simulink model "two_legged_raibert_hopper"  (R2014a)
settings: Solver=FixedStepDiscrete  StartTime=0.0  StopTime=inf  FixedStep=sample_time  RelTol=1e-3
undefined symbols (not defined in the file): boom_height, boom_mount_angle, boom_mount_to_center_diagonal, boom_mount_to_com, contact_threshold, control_start_time, desired_torso_angle, DiscIntNeverNeededParam, dt_thrust, dx_avg_desired, dx_avg_samples, dx_desired_step, extra_leg_damping, F_thrust, fcut_contact, g, i_limit_lateral, initial_dt, k_placement, k_sea, kd_flight, kd_lateral, kd_leg_angle, kd_leg_length_secondary, kd_torso, kd_virtual, ki_lateral, kp_flight_max, kp_flight_min, kp_lateral, kp_leg_angle, kp_leg_length_secondary, kp_torso, kp_virtual, l0_virtual, l_boom, l_max, l_min, l_retract, l_seg, lambda1, lambda2, lateral_offset, LEG_MTR_MAX_TORQUE, loaded_threshold, m_leg_motor, m_total_real, max_leg_angle, max_torque_lateral, min_leg_angle, sample_time, t_flight, x_limit
libraries: simulink x7
settings Model: xpc_rtwmakecfg_data=_xpcethercatlib_  BufferReuse=off  Creator=wmartin  LastModifiedBy=wmartin
settings SolverCC: EnableConcurrentExecution=on
settings DataIOCC: MaxDataPoints=1000000000  SaveFormat=StructureWithTime
settings OptimizationCC: BlockReduction=off  OptimizeBlockIOStorage=off  BufferReuse=off  GlobalBufferReuse=off  ExpressionFolding=off  ExpressionDepthLimit=2147483647  LocalBlockOutputs=off
settings DebuggingCC: UnderspecifiedInitializationDetection=Classic  StateNameClashWarn=warning
settings HardwareCC: ProdIntDivRoundTo=Zero  ProdEndianess=LittleEndian  ProdHWDeviceType=Generic->32-bit x86 compatible
settings RTWCC: SystemTargetFile=slrt.tlc  TemplateMakefile=slrt_default_tmf  Description=Simulink Real-Time  RTWVerbose=off  ProcessScript=slrt_make_rtw_hook  RTWCompilerOptimization=On
settings SimulinkRealTimeCC: GeneratePreprocessorConditionals=Disable all  EnableShiftOperators=on  RL32LogBufSizeModifier=100000000

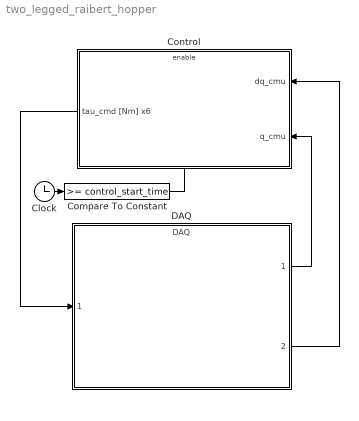
== system two_legged_raibert_hopper ==
  Clock : Clock
  Compare To Constant : simulink/Logic and Bit Operations/Compare To Constant  relop=>=  const=control_start_time  OutDataTypeStr=boolean
  Control : Subsystem
  DAQ : ModelReference  ModelNameDialog=DAQ  SimulationMode=Normal  ModelReferenceVersion=1.1405  CopyOfModelName=DAQ  DefaultDataLogging=on
  wires:
  DAQ/1 -> Control/2(q_cmu)
  DAQ/2 -> Control/1(dq_cmu)
  Clock/1 -> Compare To Constant/1
  Compare To Constant/1 -> Control/Enable
  Control/1(tau_cmd [Nm] x6) -> DAQ/1

== system two_legged_raibert_hopper/Control ==
  dq_cmu : Inport
  q_cmu : Inport  Port=2
  Enable : EnablePort  StatesWhenEnabling=reset
  Actuator Control : ModelReference  ModelNameDialog=Actuator_Control  SimulationMode=Normal  ModelReferenceVersion=1.2  CopyOfModelName=Actuator_Control  DefaultDataLogging=on
  Behavior Control : Subsystem
  tau_cmd [Nm] x6 : Outport  InitialOutput=[0 0 0 0 0 0]
  wires:
  Behavior Control/1(motor_torque_cmd) -> Actuator Control/1
  dq_cmu/1 -> Actuator Control/3, Behavior Control/1(dq_cmu)
  Actuator Control/1 -> tau_cmd [Nm] x6/1
  q_cmu/1 -> Actuator Control/2, Behavior Control/2(q_cmu)

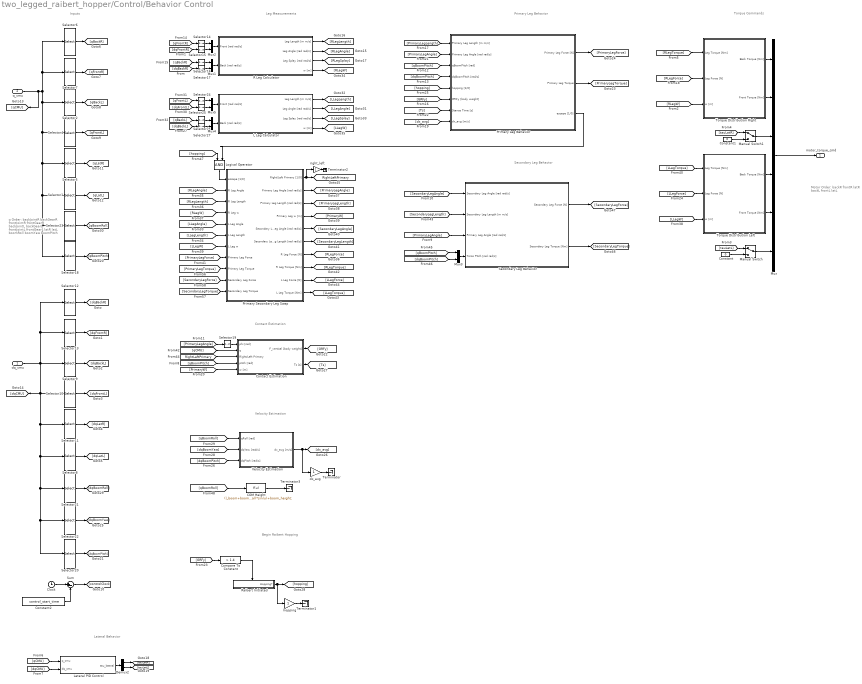
== system two_legged_raibert_hopper/Control/Behavior Control ==
  note: Motor Order:
      |
      | backR
      | frontR
      | latR
      | backL
      | frontL
      | latL
  note: q Order:
      |
      | backJointR
      | backGearR
      | frontJointR
      | frontGearR
      |
      | backJointL
      | backGearL
      | frontJointL
      | frontGearL
      |
      | latR
      | latL
      |
      | boomRoll
      | boomYaw
      | boomPitch
  note: Inputs
  note: Primary Leg Behavior
  note: Secondary Leg Behavior
  note: Torque Commands
  note: Lateral Behavior
  note: Leg Measurements
  note: Contact Estimation
  note: Velocity Estimation
  note: Begin Raibert Hopping
  dq_cmu : Inport
  q_cmu : Inport  Port=2
  COM Height : Fcn  Expr=(l_boom+boom_mount_to_center_diagonal)*sin(u)+boom_height;
  Clock : Clock
  Compare To Constant : simulink/Logic and Bit Operations/Compare To Constant  relop=>  const=1.4  OutDataTypeStr=boolean
  Constant : Constant  Value=0
  Constant1 : Constant  Value=0
  Constant2 : Constant  Value=control_start_time
  Contact Estimation : Subsystem
  Demux2 : Demux  Outputs=2
  L Leg Calculator : Subsystem
  Lateral PID Control : Subsystem
  Logical Operator : Logic  IconShape=distinctive  AllPortsSameDT=off  OutDataTypeStr=boolean
  Manual Switch : ManualSwitch
  Manual Switch1 : ManualSwitch
  Mux : Mux  Inputs=6
  Mux{1..5} (5 alike) : Mux  Inputs=2
  Primary Leg Behavior : Subsystem
  Primary Secondary Leg Swap : Subsystem
  R Leg Calculator : Subsystem
  Raibert Initiated : Subsystem
  Secondary Leg Behavior : Subsystem
  Selector1 : Selector  InputPortWidth=13  Indices=[10]
  Selector10 : Selector  InputPortWidth=13  Indices=[7 8]
  Selector11 : Selector  InputPortWidth=13  Indices=[9]
  Selector12 : Selector  InputPortWidth=13  Indices=[1 2]
  Selector13 : Selector  InputPortWidth=13  Indices=[3 4]
  Selector{14..17,19,24..27} (9 alike) : Selector  InputPortWidth=2  Indices=[1]
  Selector18 : Selector  InputPortWidth=13  Indices=[13]
  Selector2 : Selector  InputPortWidth=13  Indices=[5 6]
  Selector20 : Selector  InputPortWidth=13  Indices=[13]
  Selector21 : Selector  InputPortWidth=13  Indices=[11]
  Selector22 : Selector  InputPortWidth=13  Indices=[12]
  Selector23 : Selector  InputPortWidth=13  Indices=[11]
  Selector4 : Selector  InputPortWidth=13  Indices=[7 8]
  Selector5 : Selector  InputPortWidth=13  Indices=[9]
  Selector6 : Selector  InputPortWidth=13  Indices=[1 2]
  Selector7 : Selector  InputPortWidth=13  Indices=[3 4]
  Selector8 : Selector  InputPortWidth=13  Indices=[10]
  Selector9 : Selector  InputPortWidth=13  Indices=[5 6]
  Sum : Sum  Inputs=|+-
  Terminator{,1..3} (4 alike) : Terminator
  Torque Distribution Left : Subsystem
  Torque Distribution Right : Subsystem
  Velocity Estimation : Subsystem
  dx_avg : Gain
  hopping : Gain
  right_left : Gain
  motor_torque_cmd : Outport  OutputWhenDisabled=reset  InitialOutput=[0 0 0 0 0 0]
  tag scope: RightLeftPrimary=global
  wires:
  Lateral PID Control/1(tau_lateral) -> Demux2/1
  [dqCMU] -> Lateral PID Control/2(dq_cmu)
  [qCMU] -> Lateral PID Control/1(q_cmu)
  Sum/1 -> [controlClock]
  Selector4/1 -> [qFrontL]
  Selector2/1 -> [qBackL]
  Selector7/1 -> [qFrontR]
  Selector6/1 -> [qBackR]
  Selector1/1 -> [qLatL]
  Selector5/1 -> [qLatR]
  Constant2/1 -> Sum/2
  Clock/1 -> Sum/1
  Constant1/1 -> Manual Switch1/2
  Constant/1 -> Manual Switch/2
  Manual Switch/1 -> Mux/6
  Manual Switch1/1 -> Mux/3
  Mux/1 -> motor_torque_cmd/1
  Selector8/1 -> [dqLatL]
  Selector11/1 -> [dqLatR]
  Selector12/1 -> [dqBackR]
  Selector13/1 -> [dqFrontR]
  Selector9/1 -> [dqBackL]
  Selector10/1 -> [dqFrontL]
  [qBackR] -> Selector16/1
  [dqBackR] -> Selector17/1
  [qFrontR] -> Selector14/1
  [dqFrontR] -> Selector15/1
  Mux2/1 -> R Leg Calculator/1(Front [rad rad/s])
  Mux1/1 -> R Leg Calculator/2(Back [rad rad/s])
  R Leg Calculator/1("Leg Length [m m/s] ") -> [RLegLength]
  R Leg Calculator/2(Leg Angle [rad rad/s]) -> [RLegAngle]
  R Leg Calculator/3(Leg Splay [rad rad/s]) -> [RLegSplay]
  Torque Distribution Right/1(Back Torque [Nm]) -> Mux/1
  Torque Distribution Right/2(Front Torque [Nm]) -> Mux/2
  Demux2/1 -> [tauLatR]
  Demux2/2 -> [tauLatL]
  [tauLatR] -> Manual Switch1/1
  [tauLatL] -> Manual Switch/1
  [RLegW] -> Torque Distribution Right/3(w [m])
  Selector14/1 -> Mux2/1
  Selector15/1 -> Mux2/2
  Selector17/1 -> Mux1/2
  Selector16/1 -> Mux1/1
  [PrimaryW] -> Contact Estimation/5(w [m])
  q_cmu/1 -> Selector6/1, Selector7/1, Selector2/1, Selector4/1, Selector5/1, Selector18/1, Selector23/1, Selector1/1, [qCMU]
  Selector18/1 -> [qBoomPitch]
  [qBoomPitch] -> Contact Estimation/4(pitch [rad])
  [PrimaryLegAngle] -> Selector19/1
  Selector19/1 -> Contact Estimation/1(phi [rad])
  Contact Estimation/1(F_vertical [body weight]) -> [GRFy]
  Selector20/1 -> [dqBoomPitch]
  [RLegForce] -> Torque Distribution Right/2(Leg Force [N])
  [RLegTorque] -> Torque Distribution Right/1(Leg Torque [Nm])
  Selector22/1 -> [dqBoomYaw]
  Contact Estimation/2(Ts [s]) -> [Ts]
  [GRFy] -> Compare To Constant/1
  Raibert Initiated/1(Hopping?) -> hopping/1, [hopping]
  dq_cmu/1 -> Selector20/1, Selector22/1, Selector21/1, Selector8/1, Selector11/1, Selector10/1, [dqCMU], Selector12/1, Selector13/1, Selector9/1
  Selector21/1 -> [dqBoomRoll]
  Selector23/1 -> [qBoomRoll]
  [qBackL] -> Selector26/1
  [dqBackL] -> Selector27/1
  [qFrontL] -> Selector24/1
  [dqFrontL] -> Selector25/1
  Mux5/1 -> L Leg Calculator/1(Front [rad rad/s])
  Mux4/1 -> L Leg Calculator/2(Back [rad rad/s])
  L Leg Calculator/1("Leg Length [m m/s] ") -> [LLegLength]
  L Leg Calculator/2(Leg Angle [rad rad/s]) -> [LLegAngle]
  L Leg Calculator/3(Leg Splay [rad rad/s]) -> [LLegSplay]
  Selector24/1 -> Mux5/1
  Selector25/1 -> Mux5/2
  Selector27/1 -> Mux4/2
  Selector26/1 -> Mux4/1
  R Leg Calculator/4(w [m]) -> [RLegW]
  L Leg Calculator/4(w [m]) -> [LLegW]
  [LLegAngle] -> Primary Secondary Leg Swap/5(L Leg Angle)
  [LLegLength] -> Primary Secondary Leg Swap/6(L Leg Length)
  [LLegW] -> Primary Secondary Leg Swap/7(L Leg w)
  [RLegAngle] -> Primary Secondary Leg Swap/2(R Leg Angle)
  [RLegLength] -> Primary Secondary Leg Swap/3(R Leg Length)
  [RLegW] -> Primary Secondary Leg Swap/4(R Leg w)
  [PrimaryLegForce] -> Primary Secondary Leg Swap/8(Primary Leg Force)
  [PrimaryLegTorque] -> Primary Secondary Leg Swap/9(Primary Leg Torque)
  [SecondaryLegForce] -> Primary Secondary Leg Swap/10(Secondary Leg Force)
  [SecondaryLegTorque] -> Primary Secondary Leg Swap/11(Secondary Leg Torque)
  Primary Secondary Leg Swap/5(Secondary Leg Angle [rad rad/s]) -> [SecondaryLegAngle]
  Primary Secondary Leg Swap/6(Secondary Leg Length [rad rad/s]) -> [SecondaryLegLength]
  Primary Secondary Leg Swap/2(Primary Leg Angle [rad rad/s]) -> [PrimaryLegAngle]
  Primary Secondary Leg Swap/3(Primary Leg Length [rad rad/s]) -> [PrimaryLegLength]
  Primary Secondary Leg Swap/4(Primary Leg w [m]) -> [PrimaryW]
  Primary Secondary Leg Swap/7(R Leg Force [N]) -> [RLegForce]
  Primary Secondary Leg Swap/8(R Leg Torque [Nm]) -> [RLegTorque]
  Primary Secondary Leg Swap/9(L Leg Force [N]) -> [LLegForce]
  Primary Secondary Leg Swap/10(L Leg Torque [Nm]) -> [LLegTorque]
  Primary Leg Behavior/3(escape [1/0]) -> Logical Operator/2
  Primary Secondary Leg Swap/1(Right/Left Primary [1/0]) -> right_left/1, [RightLeftPrimary]
  [PrimaryLegLength] -> Primary Leg Behavior/1(Primary Leg Length [m m/s])
  [hopping] -> Primary Leg Behavior/5(hopping [1/0])
  [GRFy] -> Primary Leg Behavior/6(GRFy [body weight])
  [qBoomPitch] -> Primary Leg Behavior/3(qBoomPitch [rad])
  [dqBoomPitch] -> Primary Leg Behavior/4(dqBoomPitch [rad/s])
  [PrimaryLegAngle] -> Primary Leg Behavior/2(Primary Leg Angle [rad rad/s])
  [Ts] -> Primary Leg Behavior/7(Stance Time [s])
  [dx_avg] -> Primary Leg Behavior/8(dx_avg [m/s])
  Primary Leg Behavior/1(Primary Leg Force [N]) -> [PrimaryLegForce]
  Primary Leg Behavior/2(Primary Leg Torque) -> [PrimaryLegTorque]
  Velocity Estimation/1(dx_avg [m/s]) -> dx_avg/1, [dx_avg]
  [qBoomRoll] -> Velocity Estimation/1(qRoll [rad])
  [dqBoomYaw] -> Velocity Estimation/2(dqYaw [rad/s])
  [dqBoomPitch] -> Velocity Estimation/3(dqPitch [rad/s])
  dx_avg/1 -> Terminator/1
  hopping/1 -> Terminator1/1
  Torque Distribution Left/1(Back Torque [Nm]) -> Mux/4
  Torque Distribution Left/2(Front Torque [Nm]) -> Mux/5
  [LLegTorque] -> Torque Distribution Left/1(Leg Torque [Nm])
  [LLegForce] -> Torque Distribution Left/2(Leg Force [N])
  [LLegW] -> Torque Distribution Left/3(w [m])
  [qCMU] -> Contact Estimation/2(q)
  [RightLeftPrimary] -> Contact Estimation/3(Right/Left Primary)
  Secondary Leg Behavior/1(Secondary Leg Force [N]) -> [SecondaryLegForce]
  Secondary Leg Behavior/2(Secondary Leg Torque [Nm]) -> [SecondaryLegTorque]
  [PrimaryLegAngle] -> Secondary Leg Behavior/3(Primary Leg Angle [rad rad/s])
  [SecondaryLegAngle] -> Secondary Leg Behavior/1(Secondary Leg Angle [rad rad/s])
  [SecondaryLegLength] -> Secondary Leg Behavior/2(Secondary Leg Length [m m/s])
  [qBoomPitch] -> Mux3/1
  [dqBoomPitch] -> Mux3/2
  Mux3/1 -> Secondary Leg Behavior/4(Torso Pitch [rad rad/s])
  right_left/1 -> Terminator2/1
  [hopping] -> Logical Operator/1
  Logical Operator/1 -> Primary Secondary Leg Swap/1(escape [1/0])
  [qBoomRoll] -> COM Height/1
  COM Height/1 -> Terminator3/1
  Compare To Constant/1 -> Raibert Initiated/Enable

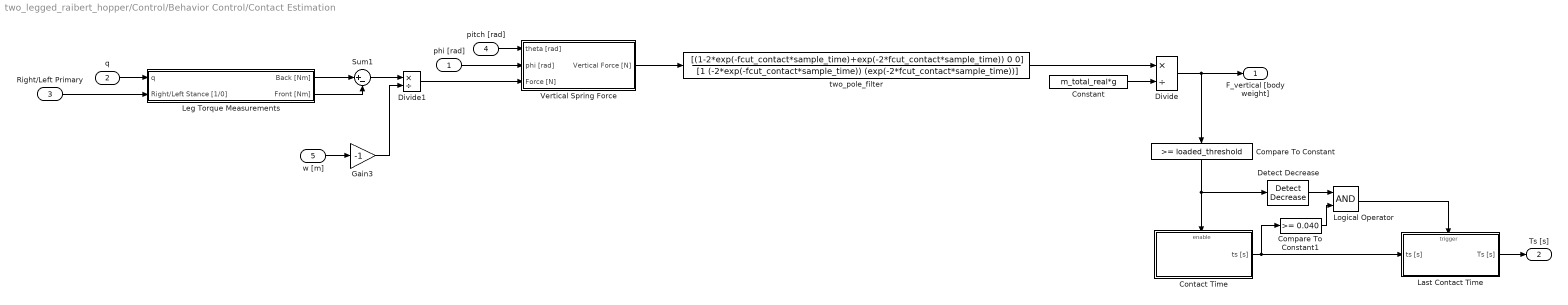
== system two_legged_raibert_hopper/Control/Behavior Control/Contact Estimation ==
  phi [rad] : Inport
  q : Inport  Port=2
  Right/Left Primary : Inport  Port=3
  pitch [rad] : Inport  Port=4
  w [m] : Inport  Port=5
  Compare To Constant : simulink/Logic and Bit Operations/Compare To Constant  relop=>=  const=loaded_threshold  OutDataTypeStr=boolean
  Compare To Constant1 : simulink/Logic and Bit Operations/Compare To Constant  relop=>=  const=0.040  OutDataTypeStr=boolean
  Constant : Constant  Value=m_total_real*g
  Contact Time : Subsystem
  Detect Decrease : simulink/Logic and Bit Operations/Detect Decrease  vinit=0.0  InputProcessing=Inherited  OutDataTypeStr=boolean
  Divide : Product  Inputs=*/
  Divide1 : Product  Inputs=*/
  Gain3 : Gain  Gain=-1
  Last Contact Time : Subsystem
  Leg Torque Measurements : Subsystem
  Logical Operator : Logic  AllPortsSameDT=off  OutDataTypeStr=boolean
  Sum1 : Sum  Inputs=|+-
  Vertical Spring Force : Subsystem
  two_pole_filter : DiscreteTransferFcn  Numerator=[(1-2*exp(-fcut_contact*sample_time)+exp(-2*fcut_contact*sample_time)) 0 0]  Denominator=[1 (-2*exp(-fcut_contact*sample_time)) (exp(-2*fcut_contact*sample_time))]  SampleTime=sample_time
  F_vertical [body weight] : Outport
  Ts [s] : Outport  Port=2
  wires:
  Vertical Spring Force/1(Vertical Force [N]) -> two_pole_filter/1
  Constant/1 -> Divide/2
  two_pole_filter/1 -> Divide/1
  q/1 -> Leg Torque Measurements/1(q)
  Leg Torque Measurements/1(Back [Nm]) -> Sum1/1
  Leg Torque Measurements/2(Front [Nm]) -> Sum1/2
  Sum1/1 -> Divide1/1
  Divide1/1 -> Vertical Spring Force/3(Force [N])
  pitch [rad]/1 -> Vertical Spring Force/1(theta [rad])
  w [m]/1 -> Gain3/1
  Gain3/1 -> Divide1/2
  phi [rad]/1 -> Vertical Spring Force/2(phi [rad])
  Last Contact Time/1(Ts [s]) -> Ts [s]/1
  Contact Time/1(ts [s]) -> Last Contact Time/1(ts [s]), Compare To Constant1/1
  Compare To Constant/1 -> Detect Decrease/1, Contact Time/Enable
  Divide/1 -> F_vertical [body weight]/1, Compare To Constant/1
  Logical Operator/1 -> Last Contact Time/Trigger
  Detect Decrease/1 -> Logical Operator/1
  Compare To Constant1/1 -> Logical Operator/2
  Right/Left Primary/1 -> Leg Torque Measurements/2(Right/Left Stance [1/0])

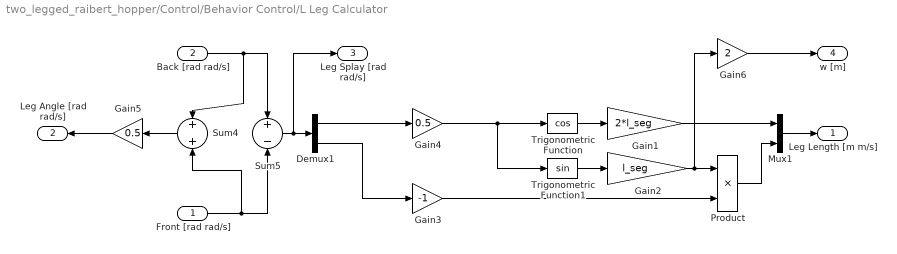
== system two_legged_raibert_hopper/Control/Behavior Control/L Leg Calculator ==
  Front [rad rad/s] : Inport
  Back [rad rad/s] : Inport  Port=2
  Demux1 : Demux  Outputs=2
  Gain1 : Gain  Gain=2*l_seg
  Gain2 : Gain  Gain=l_seg
  Gain3 : Gain  Gain=-1
  Gain4 : Gain  Gain=0.5
  Gain5 : Gain  Gain=0.5
  Gain6 : Gain  Gain=2
  Mux1 : Mux  Inputs=2
  Product : Product  RndMeth=Zero
  Sum4 : Sum  Inputs=+|+
  Sum5 : Sum  Inputs=+|-
  Trigonometric Function : Trigonometry  Operator=cos
  Trigonometric Function1 : Trigonometry
  "Leg Length [m m/s] " : Outport
  Leg Angle [rad rad/s] : Outport  Port=2
  Leg Splay [rad rad/s] : Outport  Port=3
  w [m] : Outport  Port=4
  wires:
  Gain5/1 -> Leg Angle [rad rad/s]/1
  Sum4/1 -> Gain5/1
  Mux1/1 -> "Leg Length [m m/s] "/1
  Sum5/1 -> Demux1/1, Leg Splay [rad rad/s]/1
  Gain2/1 -> Gain6/1, Product/1
  Demux1/1 -> Gain4/1
  Gain3/1 -> Product/2
  Demux1/2 -> Gain3/1
  Back [rad rad/s]/1 -> Sum5/1, Sum4/1
  Front [rad rad/s]/1 -> Sum4/2, Sum5/2
  Product/1 -> Mux1/2
  Trigonometric Function1/1 -> Gain2/1
  Gain1/1 -> Mux1/1
  Trigonometric Function/1 -> Gain1/1
  Gain4/1 -> Trigonometric Function/1, Trigonometric Function1/1
  Gain6/1 -> w [m]/1

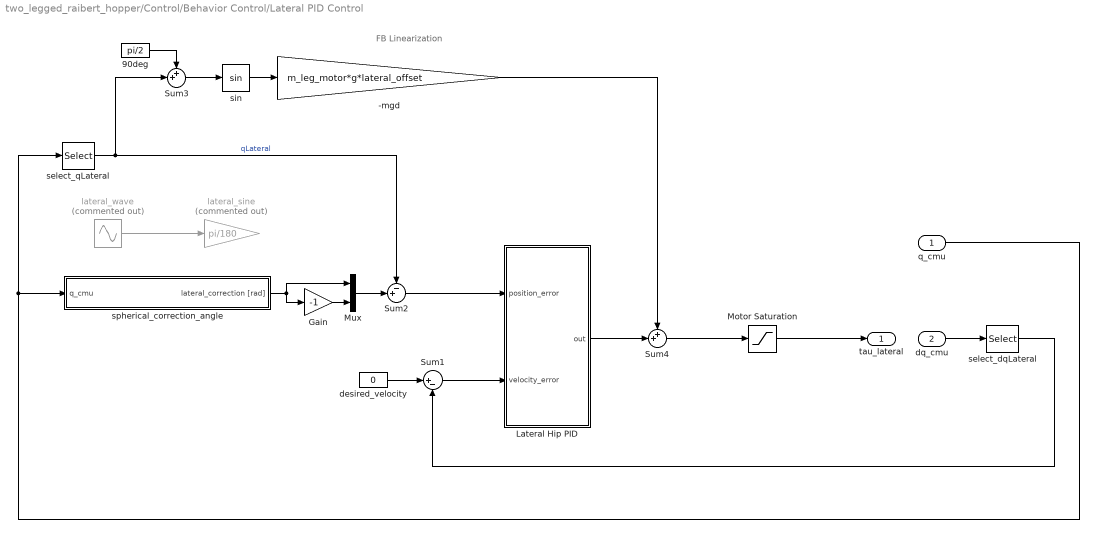
== system two_legged_raibert_hopper/Control/Behavior Control/Lateral PID Control ==
  note: FB Linearization
  q_cmu : Inport
  dq_cmu : Inport  Port=2
  -mgd : Gain  Gain=m_leg_motor*g*lateral_offset
  90deg : Constant  Value=pi/2
  Gain : Gain  Gain=-1
  Lateral Hip PID : Subsystem
  Motor Saturation : Saturate  UpperLimit=max_torque_lateral  LowerLimit=-max_torque_lateral
      settings: AttributesFormatString=Top: %<UpperLimit>\nBottom: %<LowerLimit>
  Mux : Mux  Inputs=2
  Sum1 : Sum  Inputs=|+-
  Sum2 : Sum  Inputs=-+|
  Sum3 : Sum  Inputs=++|
  Sum4 : Sum  Inputs=++|
  desired_velocity : Constant  Value=0
  lateral_sine : Gain  Commented=on  Gain=pi/180
  lateral_wave : Sin  Commented=on  Amplitude=5  Frequency=2*pi*(1/2)  SampleTime=0
  select_dqLateral : Selector  InputPortWidth=13  Indices=[9 10]
  select_qLateral : Selector  InputPortWidth=13  Indices=[9 10]
  sin : Trigonometry
  spherical_correction_angle : Subsystem
  tau_lateral : Outport
  wires:
  lateral_wave/1 -> lateral_sine/1
  Lateral Hip PID/1(out) -> Sum4/2
  Sum2/1 -> Lateral Hip PID/1(position_error)
  q_cmu/1 -> spherical_correction_angle/1(q_cmu), select_qLateral/1
  select_dqLateral/1 -> Sum1/2
  dq_cmu/1 -> select_dqLateral/1
  Sum4/1 -> Motor Saturation/1
  desired_velocity/1 -> Sum1/1
  Sum1/1 -> Lateral Hip PID/2(velocity_error)
  Gain/1 -> Mux/2
  Mux/1 -> Sum2/2
  select_qLateral/1 -> Sum3/2, Sum2/1  "qLateral"
  Motor Saturation/1 -> tau_lateral/1
  spherical_correction_angle/1(lateral_correction [rad]) -> Mux/1, Gain/1
  -mgd/1 -> Sum4/1
  Sum3/1 -> sin/1
  90deg/1 -> Sum3/1
  sin/1 -> -mgd/1

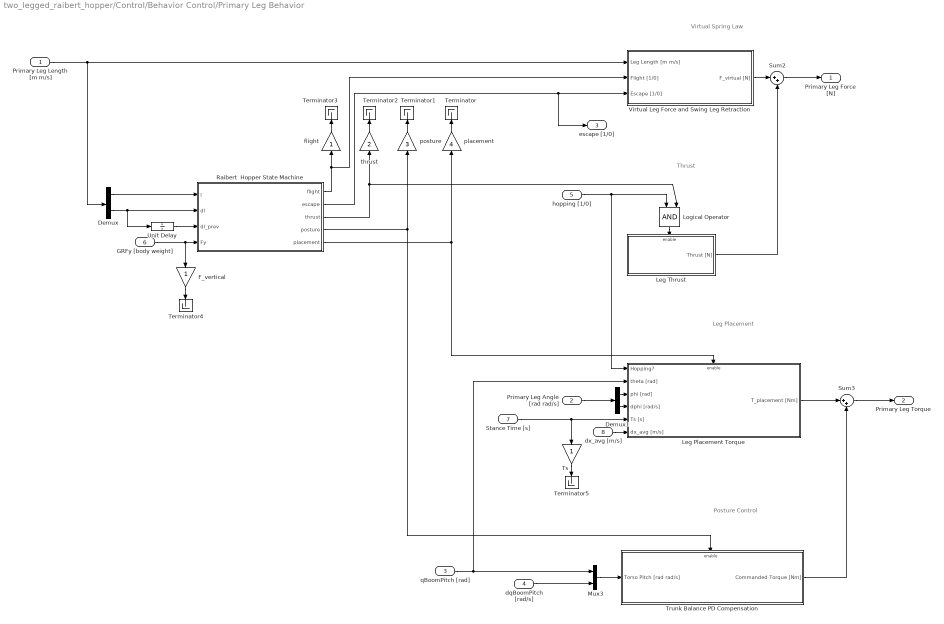
== system two_legged_raibert_hopper/Control/Behavior Control/Primary Leg Behavior ==
  note: Virtual Spring Law
  note: Thrust
  note: Posture Control
  note: Leg Placement
  Primary Leg Length [m m/s] : Inport
  Primary Leg Angle [rad rad/s] : Inport  Port=2
  qBoomPitch [rad] : Inport  Port=3
  dqBoomPitch [rad/s] : Inport  Port=4
  hopping [1/0] : Inport  Port=5
  GRFy [body weight] : Inport  Port=6
  Stance Time [s] : Inport  Port=7
  dx_avg [m/s] : Inport  Port=8
  Demux : Demux  Outputs=2
  Demux1 : Demux  Outputs=2
  F_vertical : Gain
  Leg Placement Torque : Subsystem
  Leg Thrust : Subsystem
  Logical Operator : Logic  IconShape=distinctive  AllPortsSameDT=off  OutDataTypeStr=boolean
  Mux3 : Mux  Inputs=2
  Raibert  Hopper State Machine : State Transition Table  TreatAsAtomicUnit=on
  Sum2 : Sum  Inputs=|++
  Sum3 : Sum  Inputs=|++
  Terminator{,1..5} (6 alike) : Terminator
  Trunk Balance PD Compensation : Subsystem
  Ts : Gain
  Unit Delay : UnitDelay  SampleTime=-1
  Virtual Leg Force and Swing Leg Retraction : Subsystem
  flight : Gain
  placement : Gain  Gain=4
  posture : Gain  Gain=3
  thrust : Gain  Gain=2
  Primary Leg Force [N] : Outport
  Primary Leg Torque : Outport  Port=2
  escape [1/0] : Outport  Port=3
  wires:
  Raibert  Hopper State Machine/4(posture) -> Trunk Balance PD Compensation/Enable, posture/1
  Mux3/1 -> Trunk Balance PD Compensation/1(Torso Pitch [rad rad/s])
  qBoomPitch [rad]/1 -> Mux3/1, Leg Placement Torque/2(theta [rad])
  dqBoomPitch [rad/s]/1 -> Mux3/2
  Trunk Balance PD Compensation/1(Commanded Torque [Nm]) -> Sum3/2
  Unit Delay/1 -> Raibert  Hopper State Machine/3(dl_prev)
  GRFy [body weight]/1 -> F_vertical/1, Raibert  Hopper State Machine/4(Fy)
  Demux/2 -> Unit Delay/1, Raibert  Hopper State Machine/2(dl)
  Raibert  Hopper State Machine/3(thrust) -> Logical Operator/2, thrust/1
  Leg Thrust/1(Thrust [N]) -> Sum2/2
  Sum2/1 -> Primary Leg Force [N]/1
  Raibert  Hopper State Machine/1(flight) -> flight/1, Virtual Leg Force and Swing Leg Retraction/2(Flight [1/0])
  Virtual Leg Force and Swing Leg Retraction/1(F_virtual [N]) -> Sum2/1
  Raibert  Hopper State Machine/2(escape) -> escape [1/0]/1, Virtual Leg Force and Swing Leg Retraction/3(Escape [1/0])
  Leg Placement Torque/1(T_placement [Nm]) -> Sum3/1
  Sum3/1 -> Primary Leg Torque/1
  dx_avg [m/s]/1 -> Leg Placement Torque/6(dx_avg [m/s])
  Demux1/1 -> Leg Placement Torque/3(phi [rad])
  Demux1/2 -> Leg Placement Torque/4(dphi [rad/s])
  Primary Leg Angle [rad rad/s]/1 -> Demux1/1
  Stance Time [s]/1 -> Leg Placement Torque/5(Ts [s]), Ts/1
  Raibert  Hopper State Machine/5(placement) -> Leg Placement Torque/Enable, placement/1
  Logical Operator/1 -> Leg Thrust/Enable
  placement/1 -> Terminator/1
  posture/1 -> Terminator1/1
  thrust/1 -> Terminator2/1
  Primary Leg Length [m m/s]/1 -> Demux/1, Virtual Leg Force and Swing Leg Retraction/1(Leg Length [m m/s])
  F_vertical/1 -> Terminator4/1
  flight/1 -> Terminator3/1
  Demux/1 -> Raibert  Hopper State Machine/1(l)
  Ts/1 -> Terminator5/1
  hopping [1/0]/1 -> Leg Placement Torque/1(Hopping?), Logical Operator/1

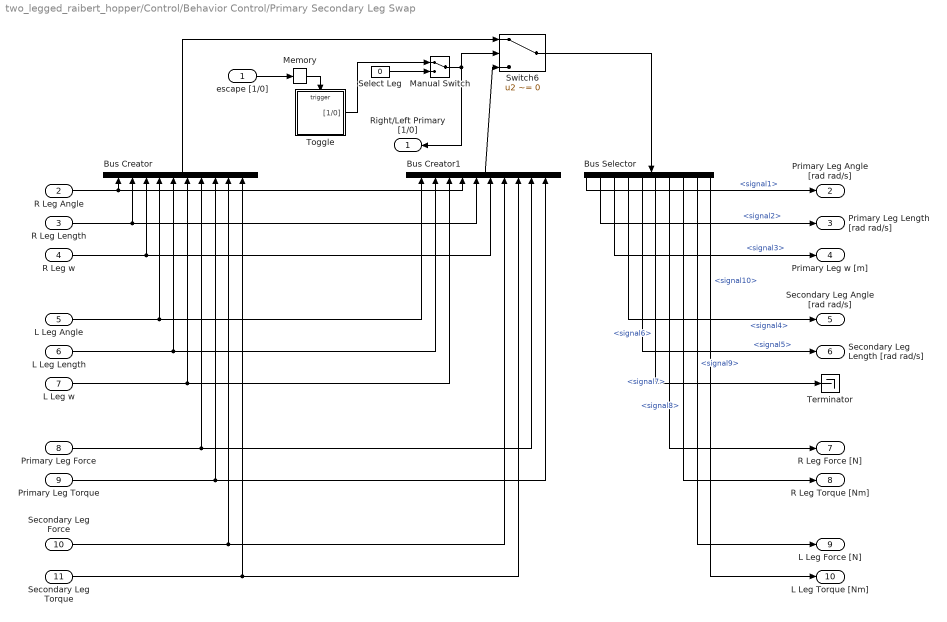
== system two_legged_raibert_hopper/Control/Behavior Control/Primary Secondary Leg Swap ==
  escape [1/0] : Inport
  R Leg Angle : Inport  Port=2
  R Leg Length : Inport  Port=3
  R Leg w : Inport  Port=4
  L Leg Angle : Inport  Port=5
  L Leg Length : Inport  Port=6
  L Leg w : Inport  Port=7
  Primary Leg Force : Inport  Port=8
  Primary Leg Torque : Inport  Port=9
  Secondary Leg Force : Inport  Port=10
  Secondary Leg Torque : Inport  Port=11
  Bus Creator : BusCreator  Inputs=10
  Bus Creator1 : BusCreator  Inputs=10
  Bus Selector : BusSelector  OutputSignals=signal1,signal2,signal3,signal4,signal5,signal6,signal7,signal8,signal9,signal10
  Manual Switch : ManualSwitch
  Memory : Memory  InheritSampleTime=on
  Select Leg : Constant  Value=0  OutDataTypeStr=boolean
  Switch6 : Switch  Criteria=u2 ~= 0  ZeroCross=off
  Terminator : Terminator
  Toggle : Subsystem
  Right/Left Primary [1/0] : Outport
  Primary Leg Angle [rad rad/s] : Outport  Port=2
  Primary Leg Length [rad rad/s] : Outport  Port=3
  Primary Leg w [m] : Outport  Port=4
  Secondary Leg Angle [rad rad/s] : Outport  Port=5
  Secondary Leg Length [rad rad/s] : Outport  Port=6
  R Leg Force [N] : Outport  Port=7
  R Leg Torque [Nm] : Outport  Port=8
  L Leg Force [N] : Outport  Port=9
  L Leg Torque [Nm] : Outport  Port=10
  wires:
  Switch6/1 -> Bus Selector/1
  Bus Creator1/1 -> Switch6/3
  Bus Creator/1 -> Switch6/1
  Primary Leg Torque/1 -> Bus Creator1/10, Bus Creator/8
  Secondary Leg Torque/1 -> Bus Creator1/8, Bus Creator/10
  Secondary Leg Force/1 -> Bus Creator1/7, Bus Creator/9
  escape [1/0]/1 -> Memory/1
  R Leg Length/1 -> Bus Creator1/5, Bus Creator/2
  L Leg w/1 -> Bus Creator/6, Bus Creator1/3
  R Leg Angle/1 -> Bus Creator1/4, Bus Creator/1
  R Leg w/1 -> Bus Creator1/6, Bus Creator/3
  Primary Leg Force/1 -> Bus Creator1/9, Bus Creator/7
  L Leg Length/1 -> Bus Creator/5, Bus Creator1/2
  L Leg Angle/1 -> Bus Creator/4, Bus Creator1/1
  Bus Selector/1 -> Primary Leg Angle [rad rad/s]/1  "<signal1>"
  Bus Selector/2 -> Primary Leg Length [rad rad/s]/1  "<signal2>"
  Bus Selector/3 -> Primary Leg w [m]/1  "<signal3>"
  Bus Selector/4 -> Secondary Leg Angle [rad rad/s]/1  "<signal4>"
  Bus Selector/5 -> Secondary Leg Length [rad rad/s]/1  "<signal5>"
  Bus Selector/6 -> Terminator/1  "<signal6>"
  Bus Selector/7 -> R Leg Force [N]/1  "<signal7>"
  Bus Selector/8 -> R Leg Torque [Nm]/1  "<signal8>"
  Bus Selector/9 -> L Leg Force [N]/1  "<signal9>"
  Bus Selector/10 -> L Leg Torque [Nm]/1  "<signal10>"
  Select Leg/1 -> Manual Switch/2
  Manual Switch/1 -> Switch6/2, Right/Left Primary [1/0]/1
  Toggle/1("[1/0]") -> Manual Switch/1
  Memory/1 -> Toggle/Trigger

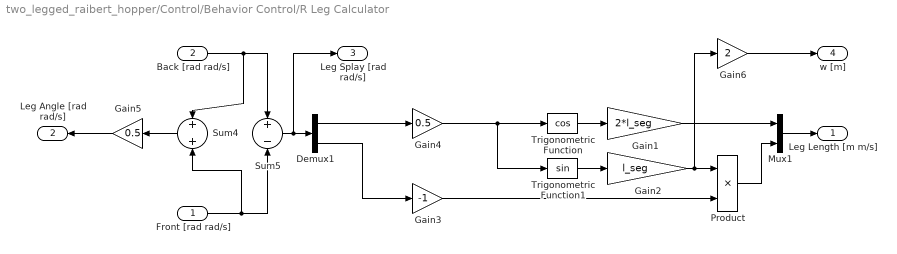
== system two_legged_raibert_hopper/Control/Behavior Control/R Leg Calculator ==
  Front [rad rad/s] : Inport
  Back [rad rad/s] : Inport  Port=2
  Demux1 : Demux  Outputs=2
  Gain1 : Gain  Gain=2*l_seg
  Gain2 : Gain  Gain=l_seg
  Gain3 : Gain  Gain=-1
  Gain4 : Gain  Gain=0.5
  Gain5 : Gain  Gain=0.5
  Gain6 : Gain  Gain=2
  Mux1 : Mux  Inputs=2
  Product : Product  RndMeth=Zero
  Sum4 : Sum  Inputs=+|+
  Sum5 : Sum  Inputs=+|-
  Trigonometric Function : Trigonometry  Operator=cos
  Trigonometric Function1 : Trigonometry
  "Leg Length [m m/s] " : Outport
  Leg Angle [rad rad/s] : Outport  Port=2
  Leg Splay [rad rad/s] : Outport  Port=3
  w [m] : Outport  Port=4
  wires:
  Gain6/1 -> w [m]/1
  Gain4/1 -> Trigonometric Function1/1, Trigonometric Function/1
  Trigonometric Function/1 -> Gain1/1
  Gain1/1 -> Mux1/1
  Trigonometric Function1/1 -> Gain2/1
  Product/1 -> Mux1/2
  Front [rad rad/s]/1 -> Sum5/2, Sum4/2
  Back [rad rad/s]/1 -> Sum4/1, Sum5/1
  Demux1/2 -> Gain3/1
  Gain3/1 -> Product/2
  Demux1/1 -> Gain4/1
  Gain2/1 -> Product/1, Gain6/1
  Sum5/1 -> Leg Splay [rad rad/s]/1, Demux1/1
  Mux1/1 -> "Leg Length [m m/s] "/1
  Sum4/1 -> Gain5/1
  Gain5/1 -> Leg Angle [rad rad/s]/1

== system two_legged_raibert_hopper/Control/Behavior Control/Raibert Initiated ==
  Enable : EnablePort  StatesWhenEnabling=reset
  Constant : Constant
  Hopping? : Outport  InitialOutput=[0]
  wires:
  Constant/1 -> Hopping?/1

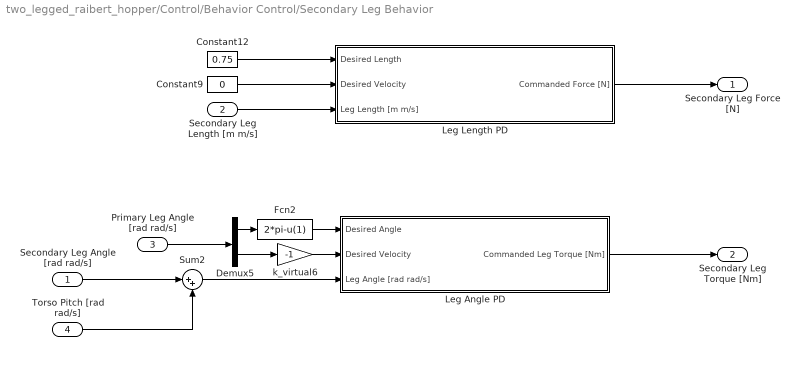
== system two_legged_raibert_hopper/Control/Behavior Control/Secondary Leg Behavior ==
  Secondary Leg Angle [rad rad/s] : Inport
  Secondary Leg Length [m m/s] : Inport  Port=2
  Primary Leg Angle [rad rad/s] : Inport  Port=3
  Torso Pitch [rad rad/s] : Inport  Port=4
  Constant12 : Constant  Value=0.75
  Constant9 : Constant  Value=0
  Demux5 : Demux  Outputs=2
  Fcn2 : Fcn  Expr=2*pi-u(1)
  Leg Angle PD : Subsystem
  Leg Length PD : Subsystem
  Sum2 : Sum  Inputs=|++
  k_virtual6 : Gain  Gain=-1
  Secondary Leg Force [N] : Outport
  Secondary Leg Torque [Nm] : Outport  Port=2
  wires:
  Constant9/1 -> Leg Length PD/2(Desired Velocity)
  Constant12/1 -> Leg Length PD/1(Desired Length)
  Secondary Leg Length [m m/s]/1 -> Leg Length PD/3(Leg Length [m m/s])
  Leg Length PD/1(Commanded Force [N]) -> Secondary Leg Force [N]/1
  Secondary Leg Angle [rad rad/s]/1 -> Sum2/1
  Torso Pitch [rad rad/s]/1 -> Sum2/2
  Sum2/1 -> Leg Angle PD/3(Leg Angle [rad rad/s])
  Fcn2/1 -> Leg Angle PD/1(Desired Angle)
  k_virtual6/1 -> Leg Angle PD/2(Desired Velocity)
  Primary Leg Angle [rad rad/s]/1 -> Demux5/1
  Demux5/1 -> Fcn2/1
  Demux5/2 -> k_virtual6/1
  Leg Angle PD/1(Commanded Leg Torque [Nm]) -> Secondary Leg Torque [Nm]/1

== system two_legged_raibert_hopper/Control/Behavior Control/Torque Distribution Left ==
  Leg Torque [Nm] : Inport
  Leg Force [N] : Inport  Port=2
  w [m] : Inport  Port=3
  Gain : Gain  Gain=0.5
  Gain1 : Gain  Gain=0.5
  Motor Torque Saturation Optimization : MATLAB Function  TreatAsAtomicUnit=on
  Product : Product  RndMeth=Zero
  Sum : Sum  Inputs=|++
  Sum1 : Sum  Inputs=+-|
  Back Torque [Nm] : Outport
  Front Torque [Nm] : Outport  Port=2
  wires:
  Gain/1 -> Motor Torque Saturation Optimization/1(x1s)
  Gain1/1 -> Motor Torque Saturation Optimization/2(x2s)
  Product/1 -> Gain1/1
  Leg Force [N]/1 -> Product/1
  Motor Torque Saturation Optimization/2(t2) -> Sum/2, Sum1/2
  w [m]/1 -> Product/2
  Motor Torque Saturation Optimization/1(t1) -> Sum1/1, Sum/1
  Sum/1 -> Front Torque [Nm]/1
  Leg Torque [Nm]/1 -> Gain/1
  Sum1/1 -> Back Torque [Nm]/1

== system two_legged_raibert_hopper/Control/Behavior Control/Torque Distribution Right ==
  Leg Torque [Nm] : Inport
  Leg Force [N] : Inport  Port=2
  w [m] : Inport  Port=3
  Gain : Gain  Gain=0.5
  Gain1 : Gain  Gain=0.5
  Motor Torque Saturation Optimization : MATLAB Function  TreatAsAtomicUnit=on
  Product : Product  RndMeth=Zero
  Sum : Sum  Inputs=|++
  Sum1 : Sum  Inputs=+-|
  Back Torque [Nm] : Outport
  Front Torque [Nm] : Outport  Port=2
  wires:
  Sum1/1 -> Back Torque [Nm]/1
  Leg Torque [Nm]/1 -> Gain/1
  Sum/1 -> Front Torque [Nm]/1
  Motor Torque Saturation Optimization/1(t1) -> Sum/1, Sum1/1
  w [m]/1 -> Product/2
  Motor Torque Saturation Optimization/2(t2) -> Sum1/2, Sum/2
  Leg Force [N]/1 -> Product/1
  Product/1 -> Gain1/1
  Gain1/1 -> Motor Torque Saturation Optimization/2(x2s)
  Gain/1 -> Motor Torque Saturation Optimization/1(x1s)

== system two_legged_raibert_hopper/Control/Behavior Control/Velocity Estimation ==
  qRoll [rad] : Inport
  dqYaw [rad/s] : Inport  Port=2
  dqPitch [rad/s] : Inport  Port=3
  Recursive Moving Average : Subsystem
  dx_from_yaw_and_roll : MATLAB Function  TreatAsAtomicUnit=on
  dx_avg [m/s] : Outport
  wires:
  Recursive Moving Average/1(dx_avg [m/s]) -> dx_avg [m/s]/1
  dx_from_yaw_and_roll/1(dx) -> Recursive Moving Average/1(dx [m/s])
  dqYaw [rad/s]/1 -> dx_from_yaw_and_roll/2(dqYaw)
  qRoll [rad]/1 -> dx_from_yaw_and_roll/1(qRoll)
  dqPitch [rad/s]/1 -> dx_from_yaw_and_roll/3(dqPitch)

== system two_legged_raibert_hopper/Control/Behavior Control/Contact Estimation/Contact Time ==
  Enable : EnablePort  StatesWhenEnabling=reset  ShowOutputPort=on
  Constant : Constant
  Discrete-Time Integrator : DiscreteIntegrator  IntegratorMethod=Accumulation: Forward Euler  gainval=sample_time  ExternalReset=rising  SampleTime=sample_time  ICPrevOutput=DiscIntNeverNeededParam  ICPrevScaledInput=DiscIntNeverNeededParam
  ts [s] : Outport  InitialOutput=[0]
  wires:
  Constant/1 -> Discrete-Time Integrator/1
  Enable/1 -> Discrete-Time Integrator/2
  Discrete-Time Integrator/1 -> ts [s]/1

== system two_legged_raibert_hopper/Control/Behavior Control/Contact Estimation/Last Contact Time ==
  ts [s] : Inport
  Trigger : TriggerPort  TriggerType=falling  PortDimensions=1
  Ts [s] : Outport  InitialOutput=[initial_dt]
  wires:
  ts [s]/1 -> Ts [s]/1

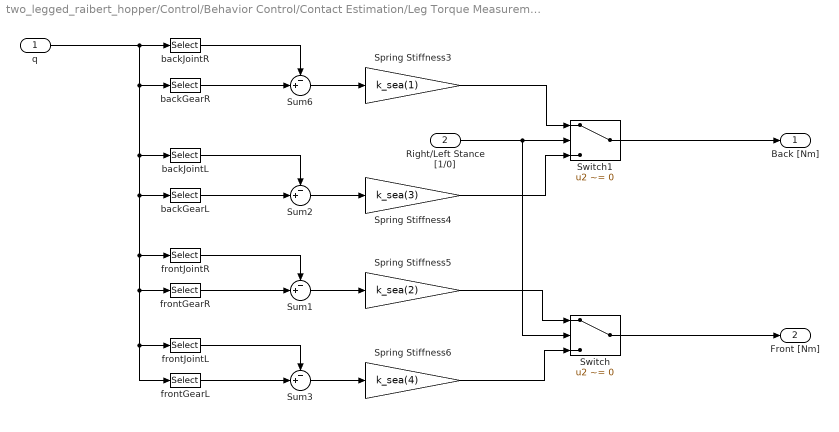
== system two_legged_raibert_hopper/Control/Behavior Control/Contact Estimation/Leg Torque Measurements ==
  q : Inport
  Right/Left Stance [1/0] : Inport  Port=2
  Spring Stiffness3 : Gain  Gain=k_sea(1)
  Spring Stiffness4 : Gain  Gain=k_sea(3)
  Spring Stiffness5 : Gain  Gain=k_sea(2)
  Spring Stiffness6 : Gain  Gain=k_sea(4)
  Sum{1..3,6} (4 alike) : Sum  Inputs=-+|
  Switch : Switch  Criteria=u2 ~= 0
  Switch1 : Switch  Criteria=u2 ~= 0
  backGearL : Selector  InputPortWidth=13  Indices=[6]
  backGearR : Selector  InputPortWidth=13  Indices=[2]
  backJointL : Selector  InputPortWidth=13  Indices=[5]
  backJointR : Selector  InputPortWidth=13  Indices=[1]
  frontGearL : Selector  InputPortWidth=13  Indices=[8]
  frontGearR : Selector  InputPortWidth=13  Indices=[4]
  frontJointL : Selector  InputPortWidth=13  Indices=[7]
  frontJointR : Selector  InputPortWidth=13  Indices=[3]
  Back [Nm] : Outport
  Front [Nm] : Outport  Port=2
  wires:
  Right/Left Stance [1/0]/1 -> Switch1/2, Switch/2
  Sum3/1 -> Spring Stiffness6/1
  Sum2/1 -> Spring Stiffness4/1
  Switch1/1 -> Back [Nm]/1
  backJointL/1 -> Sum2/1
  frontGearL/1 -> Sum3/2
  frontJointL/1 -> Sum3/1
  backGearL/1 -> Sum2/2
  Sum6/1 -> Spring Stiffness3/1
  Sum1/1 -> Spring Stiffness5/1
  Switch/1 -> Front [Nm]/1
  backJointR/1 -> Sum6/1
  frontGearR/1 -> Sum1/2
  frontJointR/1 -> Sum1/1
  backGearR/1 -> Sum6/2
  q/1 -> backGearR/1, backJointL/1, backGearL/1, frontJointR/1, frontGearR/1, frontJointL/1, frontGearL/1, backJointR/1
  Spring Stiffness3/1 -> Switch1/1
  Spring Stiffness4/1 -> Switch1/3
  Spring Stiffness5/1 -> Switch/1
  Spring Stiffness6/1 -> Switch/3

== system two_legged_raibert_hopper/Control/Behavior Control/Contact Estimation/Vertical Spring Force ==
  theta [rad] : Inport
  phi [rad] : Inport  Port=2
  Force [N] : Inport  Port=3
  Gain : Gain  Gain=-1
  Product : Product
  Sum : Sum  Inputs=++|
  Trigonometric Function : Trigonometry  Operator=cos
  Vertical Force [N] : Outport
  wires:
  Force [N]/1 -> Product/1
  phi [rad]/1 -> Sum/2
  theta [rad]/1 -> Sum/1
  Trigonometric Function/1 -> Product/2
  Product/1 -> Gain/1
  Sum/1 -> Trigonometric Function/1
  Gain/1 -> Vertical Force [N]/1

== system two_legged_raibert_hopper/Control/Behavior Control/Lateral PID Control/Lateral Hip PID ==
  position_error : Inport
  velocity_error : Inport  Port=2
  Discrete-Time Integrator : DiscreteIntegrator  IntegratorMethod=Integration: Trapezoidal  SampleTime=sample_time  LimitOutput=on  UpperSaturationLimit=i_limit_lateral  LowerSaturationLimit=-i_limit_lateral  ICPrevOutput=DiscIntNeverNeededParam  ICPrevScaledInput=DiscIntNeverNeededParam
  Sum : Sum  Inputs=+++
  kd_lateral : Gain  Description=xPCTag(1)=kd_lateral;  Gain=kd_lateral
  ki_lateral : Gain  Description=xPCTag(1)=ki_lateral;  Gain=ki_lateral
  kp_lateral : Gain  Description=xPCTag(1)=kp_lateral;  Gain=kp_lateral
  out : Outport
  wires:
  velocity_error/1 -> kd_lateral/1
  Discrete-Time Integrator/1 -> Sum/3
  ki_lateral/1 -> Discrete-Time Integrator/1
  kp_lateral/1 -> Sum/2
  position_error/1 -> ki_lateral/1, kp_lateral/1
  Sum/1 -> out/1
  kd_lateral/1 -> Sum/1

== system two_legged_raibert_hopper/Control/Behavior Control/Lateral PID Control/spherical_correction_angle ==
  q_cmu : Inport
  Selector : Selector  InputPortWidth=13  Indices=[11]
  Sum1 : Sum  Inputs=|+-
  Terminator2 : Terminator
  boom_mount_angle : Constant  Value=boom_mount_angle
  lateral_correction : Gain  Gain=180/pi
  lateral_correction [rad] : Outport
  wires:
  Sum1/1 -> lateral_correction/1, lateral_correction [rad]/1
  Selector/1 -> Sum1/1  "qBoomRoll"
  q_cmu/1 -> Selector/1
  boom_mount_angle/1 -> Sum1/2
  lateral_correction/1 -> Terminator2/1

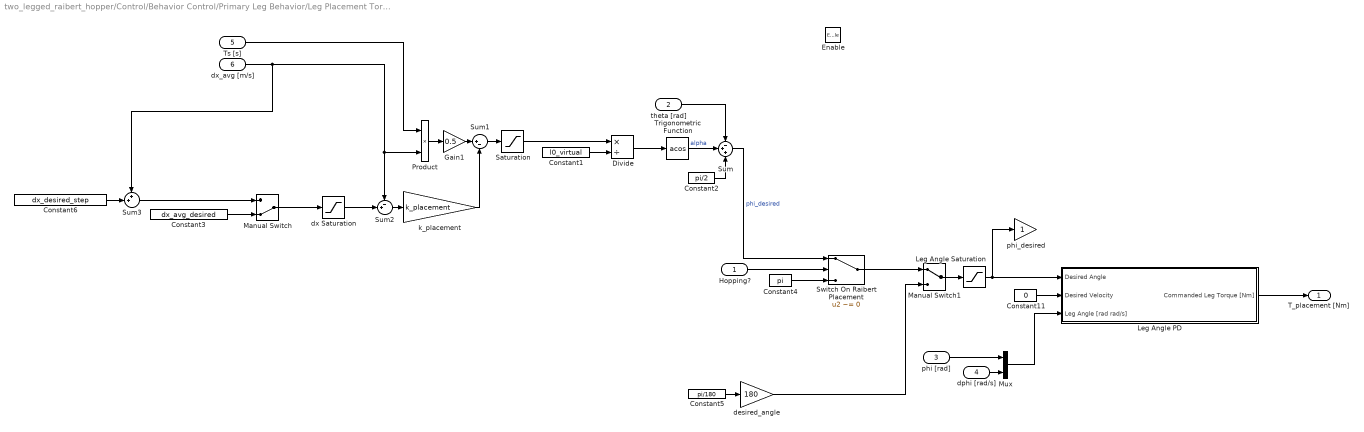
== system two_legged_raibert_hopper/Control/Behavior Control/Primary Leg Behavior/Leg Placement Torque ==
  Hopping? : Inport
  theta [rad] : Inport  Port=2
  phi [rad] : Inport  Port=3
  dphi [rad/s] : Inport  Port=4
  Ts [s] : Inport  Port=5
  dx_avg [m/s] : Inport  Port=6
  Enable : EnablePort  StatesWhenEnabling=reset
  Constant1 : Constant  Value=l0_virtual
  Constant11 : Constant  Value=0
  Constant2 : Constant  Value=pi/2
  Constant3 : Constant  Value=dx_avg_desired
  Constant4 : Constant  Value=pi
  Constant5 : Constant  Value=pi/180
  Constant6 : Constant  Value=dx_desired_step
  Divide : Product  Inputs=*/
  Gain1 : Gain  Gain=0.5
  Leg Angle PD : Subsystem
  Leg Angle Saturation : Saturate  UpperLimit=max_leg_angle  LowerLimit=min_leg_angle
      settings: AttributesFormatString=Hi: %<UpperLimit>\nLo: %<LowerLimit>
  Manual Switch : ManualSwitch  CurrentSetting=0
  Manual Switch1 : ManualSwitch
  Mux : Mux  Inputs=2
  Product : Product
  Saturation : Saturate  UpperLimit=x_limit  LowerLimit=-x_limit
      settings: AttributesFormatString=Hi: %<UpperLimit>\nLo: %<LowerLimit>
  Sum : Sum  Inputs=-++
  Sum1 : Sum  Inputs=|+-
  Sum2 : Sum  Inputs=-+|
  Sum3 : Sum  Inputs=++|
  Switch On Raibert Placement : Switch  Criteria=u2 ~= 0
  Trigonometric Function : Trigonometry  Operator=acos
  desired_angle : Gain  Gain=180
  dx Saturation : Saturate  UpperLimit=dx_avg_desired  LowerLimit=0
      settings: AttributesFormatString=Hi: %<UpperLimit>\nLo: %<LowerLimit>
  k_placement : Gain  Gain=k_placement
  phi_desired : Gain
  T_placement [Nm] : Outport  OutputWhenDisabled=reset  InitialOutput=[0]
  wires:
  Constant11/1 -> Leg Angle PD/2(Desired Velocity)
  Mux/1 -> Leg Angle PD/3(Leg Angle [rad rad/s])
  Leg Angle PD/1(Commanded Leg Torque [Nm]) -> T_placement [Nm]/1
  phi [rad]/1 -> Mux/1
  dphi [rad/s]/1 -> Mux/2
  Ts [s]/1 -> Product/1
  Product/1 -> Gain1/1
  Gain1/1 -> Sum1/1
  Saturation/1 -> Divide/1
  Constant1/1 -> Divide/2
  Trigonometric Function/1 -> Sum/2  "alpha"
  Constant2/1 -> Sum/3
  theta [rad]/1 -> Sum/1
  Sum/1 -> Switch On Raibert Placement/1  "phi_desired"
  Sum1/1 -> Saturation/1
  k_placement/1 -> Sum1/2
  Sum2/1 -> k_placement/1
  dx Saturation/1 -> Sum2/2
  Constant4/1 -> Switch On Raibert Placement/3
  Hopping?/1 -> Switch On Raibert Placement/2
  Leg Angle Saturation/1 -> phi_desired/1, Leg Angle PD/1(Desired Angle)
  Constant5/1 -> desired_angle/1
  Manual Switch/1 -> dx Saturation/1
  Constant3/1 -> Manual Switch/2
  dx_avg [m/s]/1 -> Sum3/1, Sum2/1, Product/2
  Constant6/1 -> Sum3/2
  Sum3/1 -> Manual Switch/1
  Divide/1 -> Trigonometric Function/1
  Switch On Raibert Placement/1 -> Manual Switch1/1
  desired_angle/1 -> Manual Switch1/2
  Manual Switch1/1 -> Leg Angle Saturation/1

== system two_legged_raibert_hopper/Control/Behavior Control/Primary Leg Behavior/Leg Thrust ==
  Enable : EnablePort  StatesWhenEnabling=reset  ShowOutputPort=on
  F_thrust : Gain  Gain=F_thrust
  Thrust Timer : Subsystem
  thrust period? : simulink/Logic and Bit Operations/Compare To Constant  relop=<=  const=dt_thrust  OutDataTypeStr=uint8
  Thrust [N] : Outport  OutputWhenDisabled=reset  InitialOutput=[0]
  wires:
  F_thrust/1 -> Thrust [N]/1
  Thrust Timer/1(timer [s]) -> thrust period?/1
  Enable/1 -> Thrust Timer/Enable
  thrust period?/1 -> F_thrust/1

== system two_legged_raibert_hopper/Control/Behavior Control/Primary Leg Behavior/Trunk Balance PD Compensation ==
  Torso Pitch [rad rad/s] : Inport
  Enable : EnablePort  StatesWhenEnabling=reset
  Constant2 : Constant  Value=0
  Demux : Demux  Outputs=2
  Derivative Gain : Gain  Gain=kd_torso
  Gain1 : Gain  Gain=-1
  Proportional Gain : Gain  Gain=kp_torso
  Reference Lean [rad] : Constant  Value=desired_torso_angle
  Sum1 : Sum  Inputs=|+-
  Sum4 : Sum  Inputs=|+-
  Sum5 : Sum
  Commanded Torque [Nm] : Outport  OutputWhenDisabled=reset  InitialOutput=[0]
  wires:
  Gain1/1 -> Commanded Torque [Nm]/1
  Sum1/1 -> Derivative Gain/1
  Proportional Gain/1 -> Sum5/1
  Derivative Gain/1 -> Sum5/2
  Torso Pitch [rad rad/s]/1 -> Demux/1
  Sum4/1 -> Proportional Gain/1
  Demux/1 -> Sum4/2
  Reference Lean [rad]/1 -> Sum4/1
  Constant2/1 -> Sum1/1
  Demux/2 -> Sum1/2
  Sum5/1 -> Gain1/1

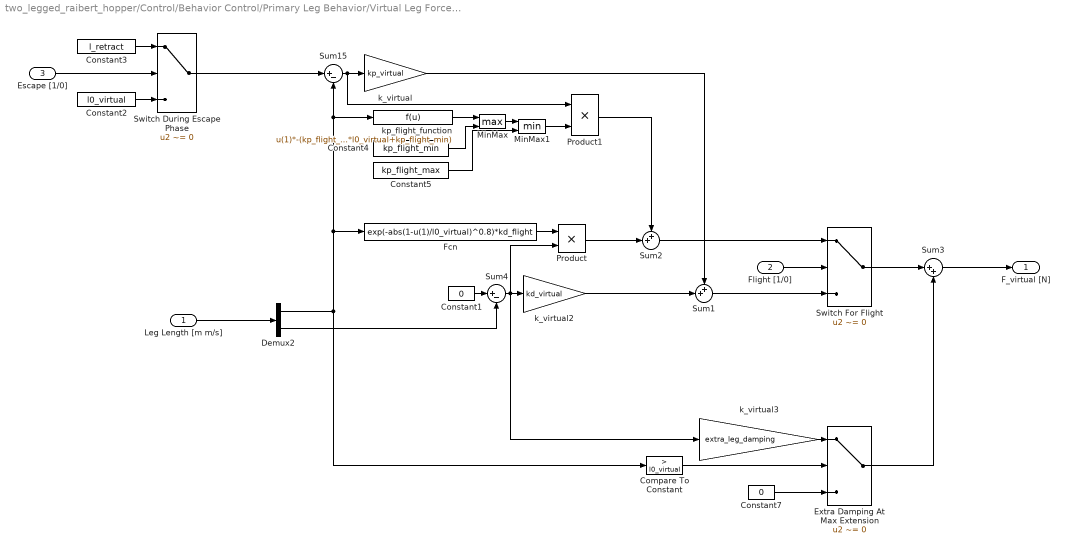
== system two_legged_raibert_hopper/Control/Behavior Control/Primary Leg Behavior/Virtual Leg Force and Swing Leg Retraction ==
  Leg Length [m m/s] : Inport
  Flight [1/0] : Inport  Port=2
  Escape [1/0] : Inport  Port=3
  Compare To Constant : simulink/Logic and Bit Operations/Compare To Constant  relop=>  const=l0_virtual  OutDataTypeStr=boolean
  Constant1 : Constant  Value=0
  Constant2 : Constant  Value=l0_virtual
  Constant3 : Constant  Value=l_retract
  Constant4 : Constant  Value=kp_flight_min
  Constant5 : Constant  Value=kp_flight_max
  Constant7 : Constant  Value=0
  Demux2 : Demux  Outputs=2
  Extra Damping At Max Extension : Switch  Criteria=u2 ~= 0
  Fcn : Fcn  Expr=exp(-abs(1-u(1)/l0_virtual)^0.8)*kd_flight
  MinMax : MinMax  Function=max  Inputs=2
  MinMax1 : MinMax  Inputs=2
  Product : Product
  Product1 : Product
  Sum1 : Sum  Inputs=++|
  Sum15 : Sum  Inputs=|+-
  Sum2 : Sum  Inputs=++|
  Sum3 : Sum  Inputs=|++
  Sum4 : Sum  Inputs=|+-
  Switch During Escape Phase : Switch  Criteria=u2 ~= 0
  Switch For Flight : Switch  Criteria=u2 ~= 0
  k_virtual : Gain  Gain=kp_virtual
  k_virtual2 : Gain  Gain=kd_virtual
  k_virtual3 : Gain  Gain=extra_leg_damping
  kp_flight_function : Fcn  Expr=u(1)*-(kp_flight_max - kp_flight_min)/(l0_virtual - l_min)+((kp_flight_max - kp_flight_min)/(l0_virtual - l_min)*l0_virtual+kp_flight_min)
  F_virtual [N] : Outport
  wires:
  Sum2/1 -> Switch For Flight/1
  Switch For Flight/1 -> Sum3/1
  Product/1 -> Sum2/2
  Constant3/1 -> Switch During Escape Phase/1
  Constant2/1 -> Switch During Escape Phase/3
  Escape [1/0]/1 -> Switch During Escape Phase/2
  Flight [1/0]/1 -> Switch For Flight/2
  k_virtual2/1 -> Sum1/2
  Sum4/1 -> k_virtual3/1, Product/2, k_virtual2/1
  k_virtual/1 -> Sum1/1
  Demux2/2 -> Sum4/2
  Constant1/1 -> Sum4/1
  Sum1/1 -> Switch For Flight/3
  Demux2/1 -> kp_flight_function/1, Sum15/2, Fcn/1, Compare To Constant/1
  Leg Length [m m/s]/1 -> Demux2/1
  Sum15/1 -> Product1/1, k_virtual/1
  Fcn/1 -> Product/1
  kp_flight_function/1 -> MinMax/1
  Product1/1 -> Sum2/1
  MinMax/1 -> MinMax1/1
  Constant4/1 -> MinMax/2
  MinMax1/1 -> Product1/2
  Constant5/1 -> MinMax1/2
  Switch During Escape Phase/1 -> Sum15/1
  Compare To Constant/1 -> Extra Damping At Max Extension/2
  Constant7/1 -> Extra Damping At Max Extension/3
  Extra Damping At Max Extension/1 -> Sum3/2
  Sum3/1 -> F_virtual [N]/1
  k_virtual3/1 -> Extra Damping At Max Extension/1

== system two_legged_raibert_hopper/Control/Behavior Control/Primary Secondary Leg Swap/Toggle ==
  Trigger : TriggerPort  TriggerType=falling  PortDimensions=1
  Logical Operator : Logic  Operator=NOT  AllPortsSameDT=off  OutDataTypeStr=boolean
  Memory : Memory  X0=1  InheritSampleTime=on
  "[1/0]" : Outport  InitialOutput=[1]
  wires:
  Memory/1 -> Logical Operator/1
  Logical Operator/1 -> Memory/1, "[1/0]"/1

== system two_legged_raibert_hopper/Control/Behavior Control/Secondary Leg Behavior/Leg Angle PD ==
  Desired Angle : Inport
  Desired Velocity : Inport  Port=2
  Leg Angle [rad rad/s] : Inport  Port=3
  Demux1 : Demux  Outputs=2
  Gain6 : Gain  Gain=kp_leg_angle
  Gain7 : Gain  Gain=kd_leg_angle
  Sum7 : Sum  Inputs=|+-
  Sum8 : Sum  Inputs=|+-
  Sum9 : Sum  Inputs=|++
  Commanded Leg Torque [Nm] : Outport
  wires:
  Leg Angle [rad rad/s]/1 -> Demux1/1
  Demux1/2 -> Sum8/2
  Gain7/1 -> Sum9/2
  Desired Angle/1 -> Sum7/1
  Sum8/1 -> Gain7/1
  Desired Velocity/1 -> Sum8/1
  Sum9/1 -> Commanded Leg Torque [Nm]/1
  Demux1/1 -> Sum7/2
  Sum7/1 -> Gain6/1
  Gain6/1 -> Sum9/1

== system two_legged_raibert_hopper/Control/Behavior Control/Secondary Leg Behavior/Leg Length PD ==
  Desired Length : Inport
  Desired Velocity : Inport  Port=2
  Leg Length [m m/s] : Inport  Port=3
  Demux1 : Demux  Outputs=2
  Sum7 : Sum  Inputs=|+-
  Sum8 : Sum  Inputs=|+-
  Sum9 : Sum
  kd_leg_length_secondary : Gain  Gain=kd_leg_length_secondary
  kp_leg_length_secondary : Gain  Gain=kp_leg_length_secondary
  Commanded Force [N] : Outport
  wires:
  kp_leg_length_secondary/1 -> Sum9/1
  Sum7/1 -> kp_leg_length_secondary/1
  Demux1/1 -> Sum7/2  "l_measured"
  Sum9/1 -> Commanded Force [N]/1
  Desired Velocity/1 -> Sum8/1
  Sum8/1 -> kd_leg_length_secondary/1
  Desired Length/1 -> Sum7/1
  kd_leg_length_secondary/1 -> Sum9/2
  Demux1/2 -> Sum8/2  "l_dot_measured"
  Leg Length [m m/s]/1 -> Demux1/1

== system two_legged_raibert_hopper/Control/Behavior Control/Velocity Estimation/Recursive Moving Average ==
  dx [m/s] : Inport
  Delay : Delay  DelayLength=dx_avg_samples  InitialCondition=0  UseCircularBuffer=on  SampleTime=sample_time
  Gain : Gain  Gain=1/dx_avg_samples
  Sum : Sum  Inputs=-++
  Unit Delay : UnitDelay  SampleTime=sample_time
  dx_avg [m/s] : Outport
  wires:
  dx [m/s]/1 -> Delay/1, Sum/2
  Sum/1 -> Gain/1, Unit Delay/1
  Delay/1 -> Sum/1
  Gain/1 -> dx_avg [m/s]/1
  Unit Delay/1 -> Sum/3

== system two_legged_raibert_hopper/Control/Behavior Control/Primary Leg Behavior/Leg Placement Torque/Leg Angle PD ==
  Desired Angle : Inport
  Desired Velocity : Inport  Port=2
  Leg Angle [rad rad/s] : Inport  Port=3
  Demux1 : Demux  Outputs=2
  Sum7 : Sum  Inputs=|+-
  Sum8 : Sum  Inputs=|+-
  Sum9 : Sum
  kd_leg_angle : Gain  Gain=kd_leg_angle
  kp_leg_angle : Gain  Gain=kp_leg_angle
  Commanded Leg Torque [Nm] : Outport
  wires:
  Leg Angle [rad rad/s]/1 -> Demux1/1
  Demux1/2 -> Sum8/2
  kd_leg_angle/1 -> Sum9/2
  Desired Angle/1 -> Sum7/1
  Sum8/1 -> kd_leg_angle/1
  Desired Velocity/1 -> Sum8/1
  Sum9/1 -> Commanded Leg Torque [Nm]/1
  Demux1/1 -> Sum7/2
  Sum7/1 -> kp_leg_angle/1
  kp_leg_angle/1 -> Sum9/1

== system two_legged_raibert_hopper/Control/Behavior Control/Primary Leg Behavior/Leg Thrust/Thrust Timer ==
  Enable : EnablePort  StatesWhenEnabling=reset  ShowOutputPort=on
  Constant : Constant
  Discrete-Time Integrator : DiscreteIntegrator  IntegratorMethod=Accumulation: Forward Euler  gainval=sample_time  ExternalReset=rising  SampleTime=sample_time  ICPrevOutput=DiscIntNeverNeededParam  ICPrevScaledInput=DiscIntNeverNeededParam
  timer [s] : Outport  InitialOutput=[0]
  wires:
  Discrete-Time Integrator/1 -> timer [s]/1
  Enable/1 -> Discrete-Time Integrator/2
  Constant/1 -> Discrete-Time Integrator/1

== stateflow chart two_legged_raibert_hopper/Control/Behavior Control/Primary Leg Behavior/Raibert  Hopper State Machine ==
  state Loading
    entry: placement = 0;
    entry: posture = 0;
    entry: thrust = 0;
    entry: flight = 0;
    entry: escape = 0;
  state Compression
    entry: placement = 0;
    entry: posture = 1;
    entry: thrust = 0;
    entry: flight = 0;
    entry: escape = 0;
  state Thrust
    entry: placement = 0;
    entry: posture = 1;
    entry: thrust = 1;
    entry: flight = 0;
    entry: escape = 0;
  state Unloading
    entry: placement = 0;
    entry: posture = 0;
    entry: thrust = 1;
    entry: flight = 0;
    entry: escape = 0;
  state Escape
    entry: placement = 0;
    entry: posture = 0;
    entry: thrust = 0;
    entry: flight = 1;
    entry: escape = 1;
  state Flight
    entry: placement = 1;
    entry: posture = 0;
    entry: thrust = 0;
    entry: flight = 1;
    entry: escape = 0;
  (junction 91) -> Loading
  Loading -> (junction 130) [order 2] : [Fy < contact_threshold]
  (junction 93) -> (junction 91)
  (junction 130) -> (junction 128)
  Loading -> Compression [order 1] : [Fy > loaded_threshold]
  (junction 115) -> Compression
  (junction 118) -> (junction 115)
  Compression -> Thrust : [dl >= 0 && dl_prev < 0]
  Thrust -> Unloading [order 1] : [Fy < loaded_threshold]
  Thrust -> (junction 102) [order 2] : [l > l_max]
  (junction 102) -> (junction 100)
  (junction 122) -> (junction 118)
  Unloading -> Escape [order 1] : [Fy < contact_threshold || l > l_max]
  Unloading -> (junction 122) [order 2] : [Fy > loaded_threshold]
  Escape -> Flight : after(t_flight,sec)
  (junction 100) -> Escape
  (default) -> Flight
  Flight -> (junction 93) : [Fy > contact_threshold]
  (junction 128) -> Flight
  data: flight output; escape output; thrust output; posture output; l input; dl input; dl_prev input; Fy input; t_flight parameter; placement output; l_max parameter; contact_threshold parameter; loaded_threshold parameter

== matlab function two_legged_raibert_hopper/Control/Behavior Control/Torque Distribution Right/Motor Torque Saturation Optimization ==
  data: x1s input; t1 output; x2s input; lambda1 parameter; lambda2 parameter; LEG_MTR_MAX_TORQUE parameter; t2 output
% Optimal leg motor torque distribution
function [t1, t2] = distribute_torque(x1s, x2s, lambda1, lambda2, LEG_MTR_MAX_TORQUE)

s = LEG_MTR_MAX_TORQUE;

% possible solutions
x1 = [                                                      x1s;
                                                            0;
                                                            s;
                                                            0;
                                                           -s;
  (lambda2*s + lambda1*x1s - lambda2*x2s)/(lambda1 + lambda2);
  (lambda1*x1s - lambda2*s + lambda2*x2s)/(lambda1 + lambda2);
  (lambda2*s + lambda1*x1s + lambda2*x2s)/(lambda1 + lambda2);
 -(lambda2*s - lambda1*x1s + lambda2*x2s)/(lambda1 + lambda2)];
 
x2 = [                                                      x2s;
                                                            s;
                                                            0;
                                                           -s;
                                                            0;
  (lambda1*s - lambda1*x1s + lambda2*x2s)/(lambda1 + lambda2);
  (lambda1*s + lambda1*x1s + lambda2*x2s)/(lambda1 + lambda2);
  (lambda1*x1s - lambda1*s + lambda2*x2s)/(lambda1 + lambda2);
 -(lambda1*s + lambda1*x1s - lambda2*x2s)/(lambda1 + lambda2)];

% test constraints
c1 = s - x1 - x2 >= 0;
c2 = s + x1 + x2 >= 0;
c3 = s - x1 + x2 >= 0;
c4 = s + x1 - x2 >= 0;
constraints = c1 & c2 & c3 & c4;

% objective function to maximize
f = -lambda1*(x1-x1s).^2-lambda2*(x2-x2s).^2;
satisfied = find(constraints);
[~,I] = max(f(satisfied));

t1 = x1(satisfied(I));
t2 = x2(satisfied(I));

== matlab function two_legged_raibert_hopper/Control/Behavior Control/Velocity Estimation/dx_from_yaw_and_roll ==
  data: qRoll input; dx output; dqYaw input; dqPitch input; l_boom parameter; boom_mount_to_center_diagonal parameter; boom_mount_to_com parameter
function dx = fcn(qRoll, dqYaw, dqPitch, l_boom, boom_mount_to_center_diagonal, boom_mount_to_com)
    dx = (l_boom+boom_mount_to_center_diagonal)*(dqYaw*cos(qRoll)) - dqPitch*boom_mount_to_com;

== matlab function two_legged_raibert_hopper/Control/Behavior Control/Torque Distribution Left/Motor Torque Saturation Optimization ==
  data: x1s input; t1 output; x2s input; lambda1 parameter; lambda2 parameter; LEG_MTR_MAX_TORQUE parameter; t2 output
% Optimal leg motor torque distribution
function [t1, t2] = distribute_torque(x1s, x2s, lambda1, lambda2, LEG_MTR_MAX_TORQUE)

s = LEG_MTR_MAX_TORQUE;

% possible solutions
x1 = [                                                      x1s;
                                                            0;
                                                            s;
                                                            0;
                                                           -s;
  (lambda2*s + lambda1*x1s - lambda2*x2s)/(lambda1 + lambda2);
  (lambda1*x1s - lambda2*s + lambda2*x2s)/(lambda1 + lambda2);
  (lambda2*s + lambda1*x1s + lambda2*x2s)/(lambda1 + lambda2);
 -(lambda2*s - lambda1*x1s + lambda2*x2s)/(lambda1 + lambda2)];
 
x2 = [                                                      x2s;
                                                            s;
                                                            0;
                                                           -s;
                                                            0;
  (lambda1*s - lambda1*x1s + lambda2*x2s)/(lambda1 + lambda2);
  (lambda1*s + lambda1*x1s + lambda2*x2s)/(lambda1 + lambda2);
  (lambda1*x1s - lambda1*s + lambda2*x2s)/(lambda1 + lambda2);
 -(lambda1*s + lambda1*x1s - lambda2*x2s)/(lambda1 + lambda2)];

% test constraints
c1 = s - x1 - x2 >= 0;
c2 = s + x1 + x2 >= 0;
c3 = s - x1 + x2 >= 0;
c4 = s + x1 - x2 >= 0;
constraints = c1 & c2 & c3 & c4;

% objective function to maximize
f = -lambda1*(x1-x1s).^2-lambda2*(x2-x2s).^2;
satisfied = find(constraints);
[~,I] = max(f(satisfied));

t1 = x1(satisfied(I));
t2 = x2(satisfied(I));
